simulink model "Sinusoidal_Steering_5_21_18"  (R2018a)
settings: Solver=FixedStepAuto  StartTime=0.0  StopTime=inf  FixedStep=.015  RelTol=1e-3  EnableMultiTasking=on
libraries: raspberrypilib x24, hdlsllib x21, simulink x11
(part 2 of 2)

== system Sinusoidal_Steering_5_21_18/Control System/Black Box/throttle_left_rear Write Message (Master --> Slave) ==
  In1 : Inport
  Bit Slice : hdlsllib/Logic and Bit Operations/Bit Slice  lidx=15  ridx=8
  Bit Slice1 : hdlsllib/Logic and Bit Operations/Bit Slice  lidx=7  ridx=0
  Display4 : Display
  Mux : Mux  Inputs=2
      settings: DisplayOption=signals
  Output : Outport
  wires:
  In1/1 -> Bit Slice1/1, Bit Slice/1
  Bit Slice1/1 -> Mux/1
  Bit Slice/1 -> Mux/2, Display4/1
  Mux/1 -> Output/1

== system Sinusoidal_Steering_5_21_18/Control System/Black Box/throttle_right_front Write Message (Master --> Slave) ==
  In1 : Inport
  Bit Slice : hdlsllib/Logic and Bit Operations/Bit Slice  lidx=15  ridx=8
  Bit Slice1 : hdlsllib/Logic and Bit Operations/Bit Slice  lidx=7  ridx=0
  Display4 : Display
  Mux : Mux  Inputs=2
      settings: DisplayOption=signals
  Output : Outport
  wires:
  Mux/1 -> Output/1
  Bit Slice/1 -> Display4/1, Mux/2
  Bit Slice1/1 -> Mux/1
  In1/1 -> Bit Slice/1, Bit Slice1/1

== system Sinusoidal_Steering_5_21_18/Control System/Black Box/throttle_right_rear Write Message (Master --> Slave) ==
  In1 : Inport
  Bit Slice : hdlsllib/Logic and Bit Operations/Bit Slice  lidx=15  ridx=8
  Bit Slice1 : hdlsllib/Logic and Bit Operations/Bit Slice  lidx=7  ridx=0
  Display4 : Display
  Mux : Mux  Inputs=2
      settings: DisplayOption=signals
  Output : Outport
  wires:
  In1/1 -> Bit Slice1/1, Bit Slice/1
  Bit Slice1/1 -> Mux/1
  Bit Slice/1 -> Mux/2, Display4/1
  Mux/1 -> Output/1
